simulink model "Sampled_HR_100t"  (R2019b)
settings: Solver=VariableStepAuto  StartTime=0.0  StopTime=10.0  RelTol=1e-3
values from neighbouring files (symbols this model uses):
  E = 3.25    [Synchronization.m]
  h = ((floor(max(100*Y))+1)*1e-2)*rand()    [Synchronization.m]    (also in bisection_function_vertical.m = (a+b)/2)
  sigma = max(X)*rand()    [Synchronization.m]    (also in bisection_function_horizontal.m = (a+b)/2; simulink_model.m = 1)
  y0 = zeros(1,nNeurons)    [Synchronization.m]
  z10 = zeros(1,nNeurons)    [Synchronization.m]
  z20 = zeros(1,nNeurons)    [Synchronization.m]
settings Model: Creator=20174245  LastModifiedBy=20174245

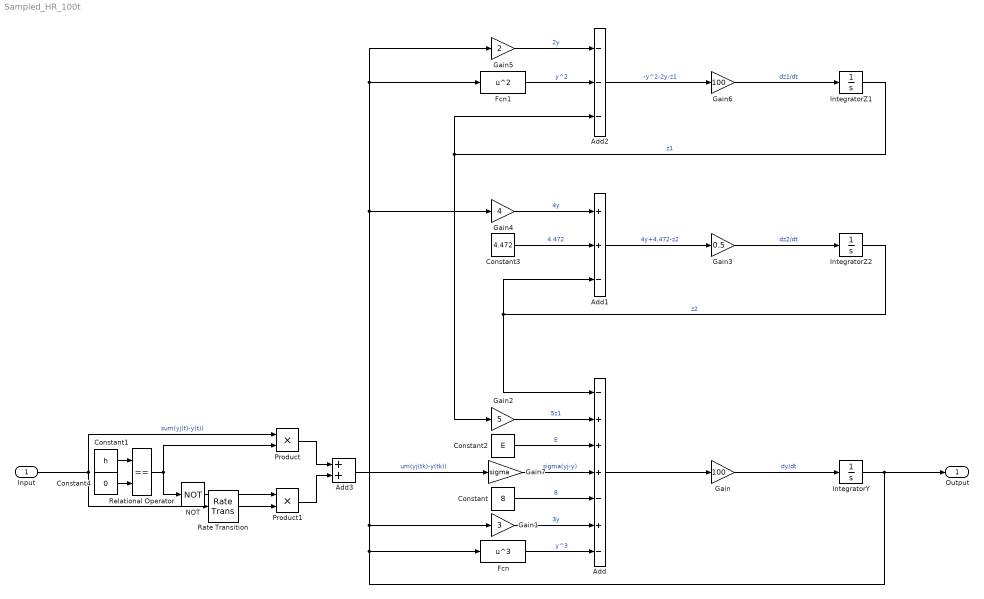
== system Sampled_HR_100t ==
  Input : Inport
  Add : Sum  Inputs=-+++-+-
  Add1 : Sum  Inputs=++-
  Add2 : Sum  Inputs=---
  Add3 : Sum
  Constant : Constant  Value=8
  Constant1 : Constant  Value=h
  Constant2 : Constant  Value=E
  Constant3 : Constant  Value=4.472
  Constant4 : Constant  Value=0
  Fcn : Fcn  Expr=u^3
  Fcn1 : Fcn  Expr=u^2
  Gain : Gain  Gain=100
  Gain1 : Gain  Gain=3
  Gain2 : Gain  Gain=5
  Gain3 : Gain  Gain=0.5
  Gain4 : Gain  Gain=4
  Gain5 : Gain  Gain=2
  Gain6 : Gain  Gain=100
  Gain7 : Gain  Gain=sigma
  IntegratorY : Integrator  InitialCondition=y0
  IntegratorZ1 : Integrator  InitialCondition=z10
  IntegratorZ2 : Integrator  InitialCondition=z20
  NOT : Logic  Operator=NOT  IconShape=distinctive  AllPortsSameDT=off  OutDataTypeStr=boolean
  Product : Product
  Product1 : Product
  Rate Transition : RateTransition  OutPortSampleTime=h
  Relational Operator : RelationalOperator  Operator===  OutDataTypeStr=boolean  RndMeth=Simplest
  Output : Outport
  wires:
  Gain6/1 -> IntegratorZ1/1  "dz1/dt"
  Add/1 -> Gain/1
  Gain/1 -> IntegratorY/1  "dy/dt"
  Gain5/1 -> Add2/1  "2y"
  Add1/1 -> Gain3/1  "4y+4.472-z2"
  Constant/1 -> Add/5  "8"
  Fcn1/1 -> Add2/2  "y^2"
  IntegratorZ1/1 -> Gain2/1, Add2/3  "z1"
  Gain2/1 -> Add/2  "5z1"
  IntegratorZ2/1 -> Add/1, Add1/3  "z2"
  Constant3/1 -> Add1/2  "4.472"
  Gain7/1 -> Add/4  "sigma(yj-y)"
  Fcn/1 -> Add/7  "y^3"
  Add2/1 -> Gain6/1  "-y^2-2y-z1"
  Gain1/1 -> Add/6  "3y"
  Constant2/1 -> Add/3  "E"
  IntegratorY/1 -> Output/1, Fcn/1, Gain1/1, Gain4/1, Fcn1/1, Gain5/1
  Gain3/1 -> IntegratorZ2/1  "dz2/dt"
  Gain4/1 -> Add1/1  "4y"
  Constant4/1 -> Relational Operator/2
  NOT/1 -> Product1/1
  Rate Transition/1 -> Product1/2
  Constant1/1 -> Relational Operator/1
  Relational Operator/1 -> NOT/1, Product/2
  Product/1 -> Add3/1
  Product1/1 -> Add3/2
  Add3/1 -> Gain7/1  "um(yj(tk)-y(tk))"
  Input/1 -> Product/1, Rate Transition/1  "sum(yj(t)-y(t))"
